simulink model "equiv_analytical"  (R2020a)
settings: Solver=FixedStepAuto  StartTime=0.0  StopTime=40  FixedStep=ts  RelTol=1e-3
InitFcn:
  | analytical_init;
  | load('eg_curve.mat');
values from neighbouring files (symbols this model uses):
  b1 = .01    (= 0.01)    [analytical_init.m]
  b2 = .001    (= 0.001)    [analytical_init.m]
  cvt_high = .81    (= 0.81)    [analytical_fitness.m]    (also in analytical_init.m)
  cvt_low = 4.31    [analytical_fitness.m]    (also in analytical_init.m)
  eg_ref = 3500    [analytical_calc.m]    (also in compare_eg_ref.m = refs(i))
  I1 = Ie + Ip    (= 0.039127939952)    [analytical_init.m]
  I2 = Is + Ig1 + Ig2/r12 + Ig3/r12 + Ig4/(r12*r34) + Ic/(r12*r34)    (= 0.170048821888)    [analytical_init.m]
  r_init = cvt_low    (= 4.31)    [analytical_init.m]
  speedVector = [1508.85099818 1518.45723596 1530.44196593 1537.65262467 1544.87011817 1563.9834899 1583.08660952 1616.48460379 1668.91395283 1709.42350202 1752.308126 1799.96340382 ... (70 elements, 70x1)]    [eg_curve.mat]
  torqueVector = [15.4893802009 16.0795925395 16.644143472 17.1317101865 17.6705997131 18.1068436155 18.4661032999 18.8510243902 19.0563156385 19.1846226686 19.2616068867 19.3899139168 ... (70 elements, 70x1)]    [eg_curve.mat]
  w1_init = 1700*(2*pi/60)    (= 178.023583703)    [analytical_init.m]
  w2_init = w1_init/r_init    (= 41.3047758013)    [analytical_init.m]
libraries: simulink x1
settings Model: Creator=Tyler  LastModifiedBy=Tyler

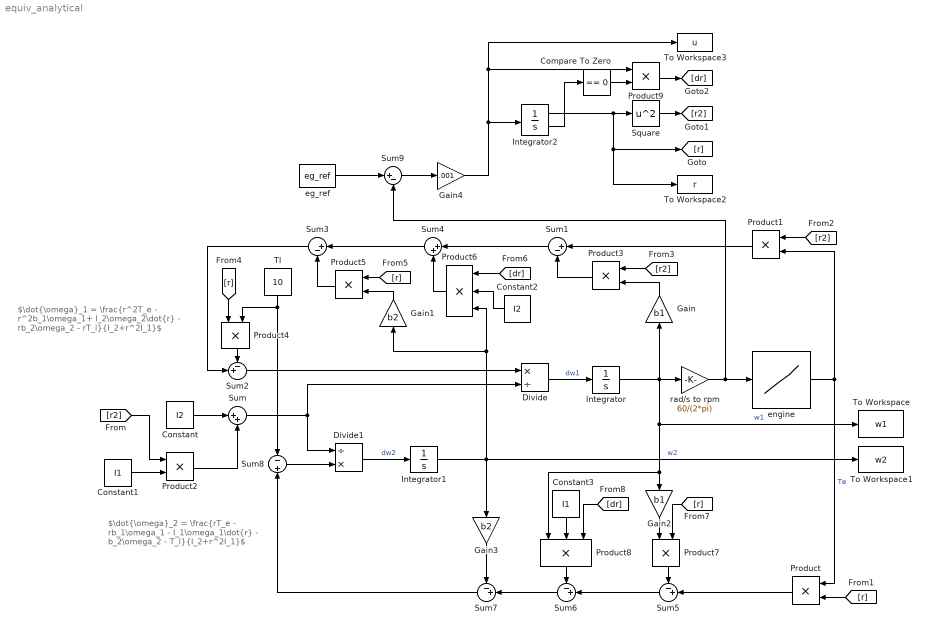
== system equiv_analytical ==
  note: $\dot{\omega}_1 = \frac{r^2T_e - r^2b_1\omega_1+ I_2\omega_2\dot{r} - rb_2\omega_2 - rT_l}{I_2+r^2I_1}$
  note: $\dot{\omega}_2 = \frac{rT_e - rb_1\omega_1 - I_1\omega_1\dot{r} - b_2\omega_2 - T_l}{I_2+r^2I_1}$
  Compare To Zero : simulink/Logic and Bit Operations/Compare To Zero  relop===  OutDataTypeStr=boolean
  Constant : Constant  Value=I2
  Constant1 : Constant  Value=I1
  Constant2 : Constant  Value=I2
  Constant3 : Constant  Value=I1
  Divide : Product  Inputs=*/
  Divide1 : Product  Inputs=/*
  Gain : Gain  Gain=b1
  Gain1 : Gain  Gain=b2
  Gain2 : Gain  Gain=b1
  Gain3 : Gain  Gain=b2
  Gain4 : Gain  Gain=.001
  Integrator : Integrator  InitialCondition=w1_init  LimitOutput=on  LowerSaturationLimit=min(speedVector)*2*pi/60
  Integrator1 : Integrator  InitialCondition=w2_init  LimitOutput=on  LowerSaturationLimit=0
  Integrator2 : Integrator  InitialCondition=r_init  LimitOutput=on  UpperSaturationLimit=cvt_low  LowerSaturationLimit=cvt_high  ShowSaturationPort=on
  Product{,1..5,7,9} (8 alike) : Product
  Product6 : Product  Inputs=3
  Product8 : Product  Inputs=3
  Square : Math  Operator=square  SaturateOnIntegerOverflow=on
  Sum : Sum  Inputs=|++
  Sum1 : Sum  Inputs=|+-
  Sum{2,5..7} (4 alike) : Sum  Inputs=-+|
  Sum3 : Sum  Inputs=|+-
  Sum4 : Sum  Inputs=|++
  Sum8 : Sum  Inputs=-|+
  Sum9 : Sum  Inputs=|+-
  Tl : Constant  Value=10
  To Workspace : ToWorkspace  VariableName=w1  SaveFormat=Timeseries  SampleTime=-1
  To Workspace1 : ToWorkspace  VariableName=w2  SaveFormat=Timeseries  SampleTime=-1
  To Workspace2 : ToWorkspace  VariableName=r  SaveFormat=Timeseries  SampleTime=-1
  To Workspace3 : ToWorkspace  VariableName=u  SaveFormat=Timeseries  SampleTime=-1
  eg_ref : Constant  Value=eg_ref
  engine : Lookup_n-D  NumberOfTableDimensions=1  BreakpointsForDimension1=speedVector  Table=torqueVector  InternalRulePriority=Speed  RndMeth=Simplest  InputSameDT=on
  rad/s to rpm : Gain  Gain=60/(2*pi)
  wires:
  Integrator2/1 -> To Workspace2/1, [r], Square/1
  Integrator/1 -> Product8/1, Gain2/1, To Workspace/1, rad/s to rpm/1, Gain/1  "w1"
  Integrator1/1 -> To Workspace1/1, Gain1/1, Product6/3, Gain3/1  "w2"
  Divide/1 -> Integrator/1  "dw1"
  Divide1/1 -> Integrator1/1  "dw2"
  engine/1 -> Product/1, Product1/2  "Te"
  Sum/1 -> Divide1/1, Divide/2
  Square/1 -> [r2]
  [r2] -> Product2/1
  Constant1/1 -> Product2/2
  [r2] -> Product1/1
  [r2] -> Product3/1
  Gain/1 -> Product3/2
  Product1/1 -> Sum1/1
  Product3/1 -> Sum1/2
  Tl/1 -> Product4/2, Sum8/1
  [r] -> Product4/1
  Product5/1 -> Sum3/2
  [r] -> Product5/1
  Gain1/1 -> Product5/2
  Product6/1 -> Sum4/2
  [dr] -> Product6/1
  Sum2/1 -> Divide/1
  Product/1 -> Sum5/2
  Gain2/1 -> Product7/1
  [r] -> Product7/2
  Product7/1 -> Sum5/1
  Sum5/1 -> Sum6/2
  Sum6/1 -> Sum7/2
  Gain3/1 -> Sum7/1
  Product8/1 -> Sum6/1
  [dr] -> Product8/3
  [r] -> Product/2
  Constant3/1 -> Product8/2
  Sum7/1 -> Sum8/2
  Sum8/1 -> Divide1/2
  Product4/1 -> Sum2/1
  Constant/1 -> Sum/1
  Product2/1 -> Sum/2
  Sum1/1 -> Sum4/1
  Sum4/1 -> Sum3/1
  Sum3/1 -> Sum2/2
  Constant2/1 -> Product6/2
  rad/s to rpm/1 -> Sum9/2, engine/1
  eg_ref/1 -> Sum9/1
  Sum9/1 -> Gain4/1
  Gain4/1 -> Product9/1, To Workspace3/1, Integrator2/1
  Product9/1 -> [dr]
  Compare To Zero/1 -> Product9/2
  Integrator2/2 -> Compare To Zero/1
